simulink model "wk2_3"  (R2020b)
settings: Solver=VariableStepAuto  StartTime=0.0  StopTime=120  RelTol=1e-3
PreLoadFcn:
  | clear all;
  | close all;
  | clc;
  | m=1000;
  | b=50;
  | u=500;
settings Model: DataDictionary=dd.sldd  Creator=hp  LastModifiedBy=ASUS

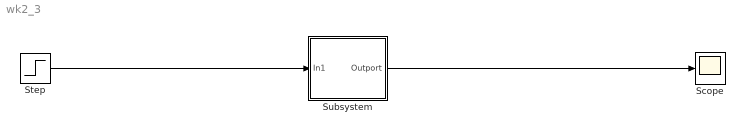
== system wk2_3 ==
  Scope : Scope
  Step : Step  Time=0  After=u  SampleTime=0
  Subsystem : Subsystem
  wires:
  Step/1 -> Subsystem/1(In1)
  Subsystem/1(Outport) -> Scope/1

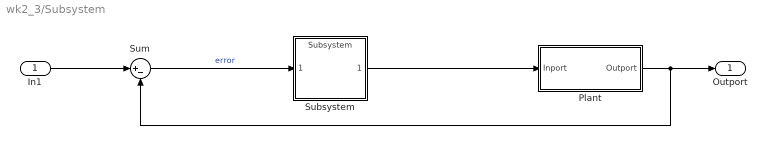
== system wk2_3/Subsystem ==
  In1 : Inport
  Plant : Subsystem
  Subsystem : ModelReference  ModelNameDialog=Subsystem  SimulationMode=Normal  ModelReferenceVersion=1.12
  Sum : Sum  Inputs=|+-
  Outport : Outport
  wires:
  Plant/1(Outport) -> Outport/1, Sum/2
  In1/1 -> Sum/1
  Sum/1 -> Subsystem/1  "error"
  Subsystem/1 -> Plant/1(Inport)

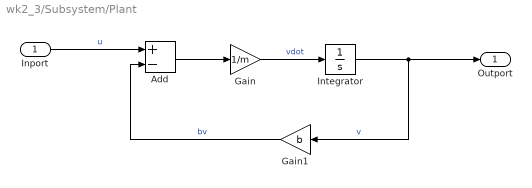
== system wk2_3/Subsystem/Plant ==
  Inport : Inport
  Add : Sum  Inputs=+-
  Gain : Gain  Gain=1/m
  Gain1 : Gain  Gain=b
  Integrator : Integrator
  Outport : Outport
  wires:
  Gain1/1 -> Add/2  "bv"
  Add/1 -> Gain/1
  Integrator/1 -> Outport/1, Gain1/1  "v"
  Gain/1 -> Integrator/1  "vdot"
  Inport/1 -> Add/1  "u"
